simulink model "Household"  (R2019b)
settings: Solver=VariableStepAuto  StartTime=0.0  StopTime=86400  RelTol=1e-3
settings Model: Creator=jorge  LastModifiedBy=jorge

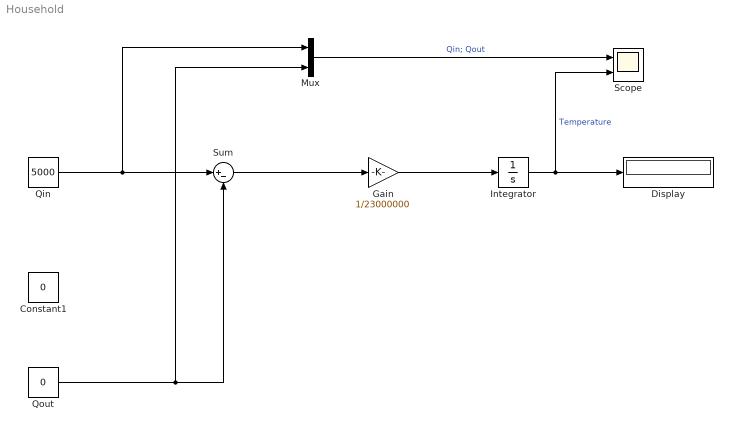
== system Household ==
  Constant1 : Constant  Value=0
  Display : Display
  Gain : Gain  Gain=1/23000000
  Integrator : Integrator  InitialCondition=20
  Mux : Mux  Inputs=2
  Qin : Constant  Value=5000
  Qout : Constant  Value=0
  Scope : Scope  NumInputPorts=2
  Sum : Sum  Inputs=|+-
  wires:
  Gain/1 -> Integrator/1
  Sum/1 -> Gain/1
  Qin/1 -> Mux/1, Sum/1
  Mux/1 -> Scope/1  "Qin; Qout"
  Integrator/1 -> Scope/2, Display/1  "Temperature"
  Qout/1 -> Mux/2, Sum/2
